simulink model "CarModel"  (R2016b)
settings: Solver=VariableStepAuto  StartTime=0.0  StopTime=10  FixedStep=0.00001  MaxStep=0.023  RelTol=1e-3
undefined symbols (not defined in the file or in its folder): sigbuilder_block
settings Model: Creator=Laurens  LastModifiedBy=Laurens

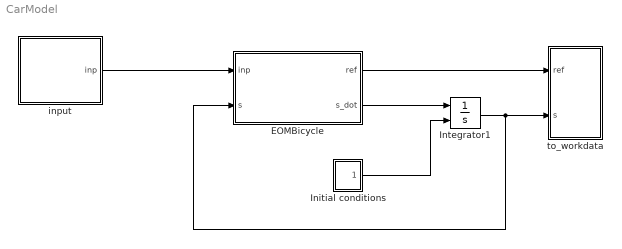
== system CarModel ==
  EOMBicycle : MATLAB Function  TreatAsAtomicUnit=on
  Initial conditions : Subsystem
  Integrator1 : Integrator  InitialConditionSource=external
  input : Subsystem
  to_workdata : Subsystem
  wires:
  EOMBicycle/2(s_dot) -> Integrator1/1
  Initial conditions/1(s0) -> Integrator1/2
  input/1(inp) -> EOMBicycle/1(inp)
  Integrator1/1 -> to_workdata/2(s), EOMBicycle/2(s)
  EOMBicycle/1(ref) -> to_workdata/1(ref)

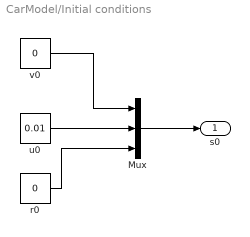
== system CarModel/Initial conditions ==
  Mux : Mux  Inputs=3
  r0 : Constant  Value=0
  u0 : Constant  Value=0.01
  v0 : Constant  Value=0
  s0 : Outport
  wires:
  v0/1 -> Mux/1
  u0/1 -> Mux/2
  r0/1 -> Mux/3
  Mux/1 -> s0/1

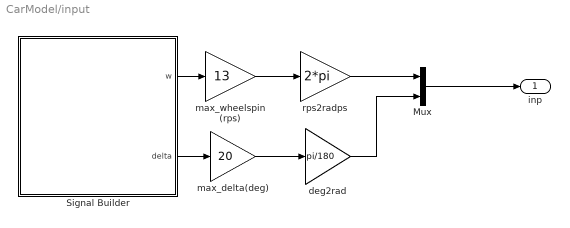
== system CarModel/input ==
  Mux : Mux  Inputs=2
  Signal Builder : Subsystem  Tag=STV Subsys  LoadFcn=sigbuilder_block('load');  StartFcn=sigbuilder_block('start');  StopFcn=sigbuilder_block('stop');  ClipboardFcn=sigbuilder_block('clipboard');  mask(Sigbuilder block){tuvar=[0:10]}
      mask help: Simulink:masks:SigbuilderBlock_MD
      mask init:
      | if ~strcmp(get_param(bdroot(gcbh),'SimulationStatus'),'stopped') tuvar = sigbuilder_block('maskInit'); end
      settings: CopyFcn=sigbuilder_block('copy');  DeleteFcn=sigbuilder_block('delete');  ModelCloseFcn=sigbuilder_block('modelClose');  PreSaveFcn=sigbuilder_block('preSave');  PauseFcn=sigbuilder_block('pause');  ContinueFcn=sigbuilder_block('continue');  NameChangeFcn=sigbuilder_block('namechange');  OpenFcn=sigbuilder_block('open',[5.4 34.2 1141.2 523.8 ]);  CloseFcn=sigbuilder_block('close');
      mask Display: plot(0, 0, 100, 100,[2, 2, 32, 32, 2], [68, 8, 8, 68, 68],[32, 2], [38, 38], [32, 19, 2],[53, 60, 44], [32, 17, 17, 2],[16, 16, 31, 31]);txt = getActiveGroup(gcbh);text(2, 100, txt,'verticalAlignment', 'top');
  deg2rad : Gain  Gain=pi/180
  max_delta(deg) : Gain  Gain=20
  max_wheelspin (rps) : Gain  Gain=13
  rps2radps : Gain  Gain=2*pi
  inp : Outport
  wires:
  max_delta(deg)/1 -> deg2rad/1
  max_wheelspin (rps)/1 -> rps2radps/1
  deg2rad/1 -> Mux/2
  rps2radps/1 -> Mux/1
  Signal Builder/1(w) -> max_wheelspin (rps)/1
  Mux/1 -> inp/1
  Signal Builder/2(delta) -> max_delta(deg)/1

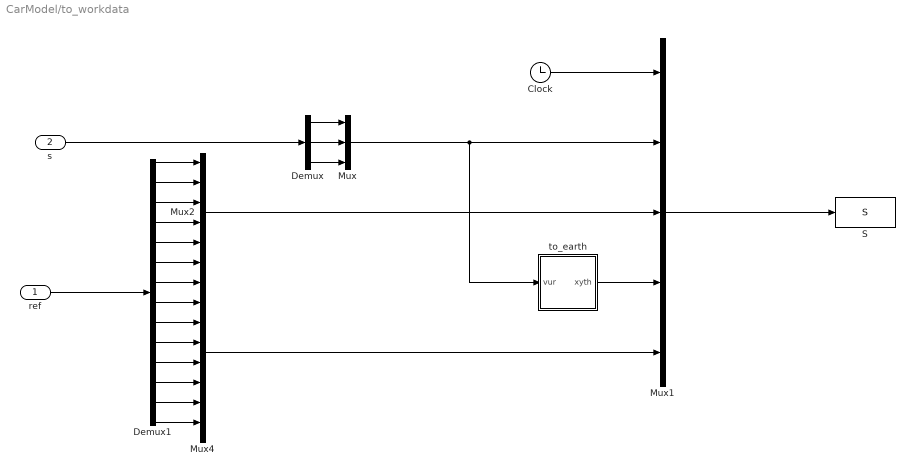
== system CarModel/to_workdata ==
  ref : Inport
  s : Inport  Port=2
  Clock : Clock
  Demux : Demux  Outputs=3
  Demux1 : Demux  Outputs=14
  Mux : Mux  Inputs=3
  Mux1 : Mux  Inputs=5
  Mux2 : Mux  Inputs=6
  Mux4 : Mux  Inputs=8
  S : ToWorkspace  VariableName=S  SampleTime=-1
  to_earth : Subsystem
  wires:
  Clock/1 -> Mux1/1
  ref/1 -> Demux1/1
  Mux2/1 -> Mux1/3
  Demux1/1 -> Mux2/1
  Demux1/2 -> Mux2/2
  Demux1/3 -> Mux2/3
  to_earth/1(xyth) -> Mux1/4
  Demux1/7 -> Mux4/1
  Demux1/8 -> Mux4/2
  Demux1/9 -> Mux4/3
  Demux1/10 -> Mux4/4
  Demux1/11 -> Mux4/5
  Demux1/12 -> Mux4/6
  Demux1/13 -> Mux4/7
  Demux1/14 -> Mux4/8
  Demux1/4 -> Mux2/4
  Demux1/5 -> Mux2/5
  Demux1/6 -> Mux2/6
  Mux4/1 -> Mux1/5
  Mux1/1 -> S/1
  Demux/1 -> Mux/1
  Demux/2 -> Mux/2
  Demux/3 -> Mux/3
  Mux/1 -> to_earth/1(vur), Mux1/2
  s/1 -> Demux/1

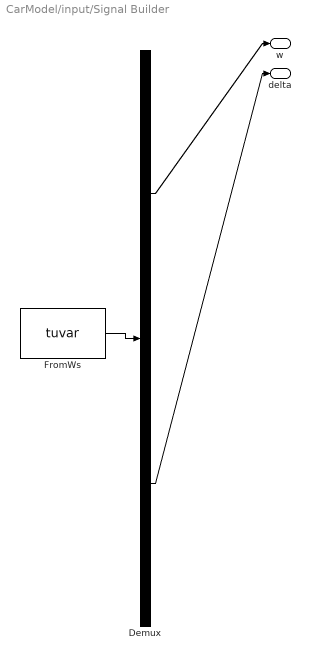
== system CarModel/input/Signal Builder ==
  Demux : Demux  Tag=STV Demux  Outputs=2
  FromWs : FromWorkspace  Tag=STV FromWs  VariableName=tuvar  SampleTime=0
      SigBuilderData=|
      | common.afterFinalStr = 'Extrapolate'
      | common.sampleTime = 0
      | dataSet.timeRange = [0 10]
      | dataSet.name = 'Group 1'
      | sbobj.Groups.Name = 'Group 1'
      | sbobj.Groups.Signals(1).Name = 'w'
      | sbobj.Groups.Signals(1).XData = [0 10]
      | sbobj.Groups.Signals(1).YData = [1 1]
      | sbobj.Groups.Signals(2).Name = 'delta'
      | sbobj.Groups.Signals(2).XData = [0 2.5 3 4.52 5.01 5.98 10]
      | sbobj.Groups.Signals(2).YData = [0 0 0.5 0.5 -0.5 -0.5 -0.5]
  w : Outport  Tag=STV Outport
  delta : Outport  Tag=STV Outport  Port=2
  wires:
  FromWs/1 -> Demux/1
  Demux/1 -> w/1
  Demux/2 -> delta/1

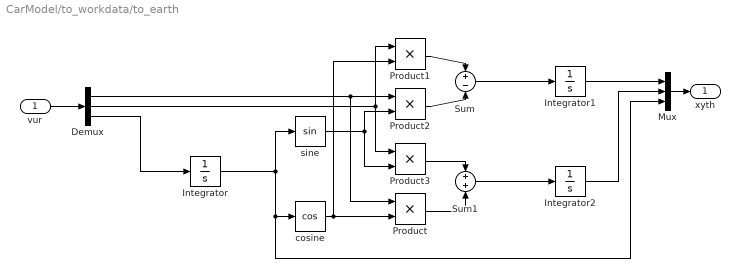
== system CarModel/to_workdata/to_earth ==
  vur : Inport
  Demux : Demux  Outputs=3
  Integrator : Integrator
  Integrator1 : Integrator
  Integrator2 : Integrator
  Mux : Mux  Inputs=3
  Product{,1..3} (4 alike) : Product
  Sum : Sum  Inputs=+-
  Sum1 : Sum
  cosine : Trigonometry  Operator=cos
  "sine " : Trigonometry
  xyth : Outport
  wires:
  Demux/3 -> Integrator/1
  Product1/1 -> Sum/1
  Product2/1 -> Sum/2
  Product3/1 -> Sum1/1
  Product/1 -> Sum1/2
  Integrator/1 -> Mux/3, cosine/1, "sine "/1
  "sine "/1 -> Product3/2, Product2/2
  Demux/1 -> Product/1, Product2/1
  cosine/1 -> Product1/2, Product/2
  Demux/2 -> Product1/1, Product3/1
  Sum/1 -> Integrator1/1
  Sum1/1 -> Integrator2/1
  Integrator1/1 -> Mux/1
  Integrator2/1 -> Mux/2
  vur/1 -> Demux/1
  Mux/1 -> xyth/1

== matlab function CarModel/EOMBicycle ==
  data: ref output; inp input; s input; s_dot output
function [ref, s_dot] =  EOMBicycle(inp, s)
%% Trivia
% Author            Laurens Znidarsic
% Version           6
% Last edit         10-07-2017
% Last edit by      Laurens Znidarsic

%% Description 
% Represents the equations of motion for an RC car test rig.

%% unpack state and input vectors
wr = inp(1);
delta = inp(2);
v = s(1);
u = s(2);
r = s(3);


%% Car parameters
Ckf  = 200;                           % [N]      Front longitudinal tire stifness
Ckr = 200;                            % [N]      Rear longitudinal tire stifness
Caf = 120;                            % [N/rad]  Front Cornering stiffness
Car = 120;                            % [N/rad]  Rear Cornering stifness
lf  = 0.167;                         % [m]      Distance from front axle to CoG
lr  = 0.167;                         % [m]      Distance from rear axle to CoG
m   = 3.2;                           % [kg]     Car mass
Iz  = 0.048875;                      % [kg*m^2] Inertia of the car
rw  = [0.048, 0.048];                % [m]      Radius of the wheels
Jw  = [0.000100359, 0.000100359];    % [kg*m^2] Inertia of the wheels
mu  = 0.6;                           % [-]      Road friction coefficient 
g = 9.81;                            % [m/s^2]  Gravity
u_min = 0.01;                        % [m/s]    Velocity threshhold

%% Slip

% Calculate wheelcentervelocity and create thresholds to avoid
% singularities 

vxw = cos(delta)*u + sin(delta)*(v + r*lf);     % Front wheelcentervelocity
u_thr = Threshold(u, u_min);                    % Longitudinal velocity threshold
vxw_thr = Threshold(vxw, u_min);                % Front wheelcentervelocity threshold
wf = (wr/u_thr)*vxw;                            % Enlarge front wheelspin as result of corners (beunoplossing!)
vwf = Threshold(wf*rw(1), u_min);               % Threshold front wheelspin 
vwr = Threshold(wr*rw(2), u_min);               % Threshold rear wheelspin

kappa = zeros(2,1);                             % kappa = [kappa_f;kappa_r]
kappa(1) = (wf*rw(1) - vxw)/absmax(vwf,vxw_thr);% slipratio rearwheel
kappa(2) = (wr*rw(2) - u)/absmax(vwr,u_thr);    % slipratio frontwheel

alpha = zeros(2,1);                             % alpha = [alpha_f;alpha_r]
alpha(1) = delta -  revtan(v+lf*r, u);          % slipangle frontwheel
alpha(2) = - revtan(v-lr*r, u);                 % slipangle rearwheel


%% Tyre model

% Linear tire model
Fxw = [Ckf*kappa(1); Ckr*kappa(2)];
Fyw = [Caf*alpha(1); Car*alpha(2)];

%% To car frame
%For coordinate system, see BSc paper 
Fxf = cos(delta)*Fxw(1) - sin(delta)*Fyw(1);
Fyf = sin(delta)*Fxw(1) + cos(delta)*Fyw(1);
Fxr = Fxw(2);
Fyr = Fyw(2);

%% Dynamics (Eq. of motion)

% Equations of motion
v_dot = (Fyf + Fyr)/m - u*r;                         % F = m*a
r_dot = (lf*Fyf - lr*Fyr)/Iz;                        % M = I*alpha
u_dot = (Fxf + Fxr)/m + v*r;                         % F = m*a

s_dot = [v_dot u_dot r_dot];                         % to store velocities
ref = [v_dot u_dot r_dot wf wr delta Fxf Fxr Fyf Fyr kappa.' alpha.'];  % to store other variables
      

end
